simulink model "lab_cc_controlador"  (R2015a)
settings: Solver=ode45  StartTime=0.0  StopTime=40  RelTol=1e-6
values from neighbouring files (symbols this model uses):
  A = [2.8883370741 1 0 0 0 -2.75968400411 0 1 0 0 0.525095601237 0 ... (25 elements, 5x5)]    [model_matrix_data424.mat]
  B = [1 0 0 0 0]    [model_matrix_data424.mat]
  C = [-0.0748175001742 0.149096420272 0 0 0]    [model_matrix_data424.mat]
  D = 0    [model_matrix_data424.mat]
  N = Ny+K*Nx    [lab4script.m]    (also in test_different_R.m; teste_sistema_real.m)
  Ts = 0.02    [lab4script.m]    (also in test_different_R.m; teste_sistema_real.m)
undefined symbols (not defined in the file or in its folder): K, M
settings Model: Creator=Margarida  LastModifiedBy=Margarida

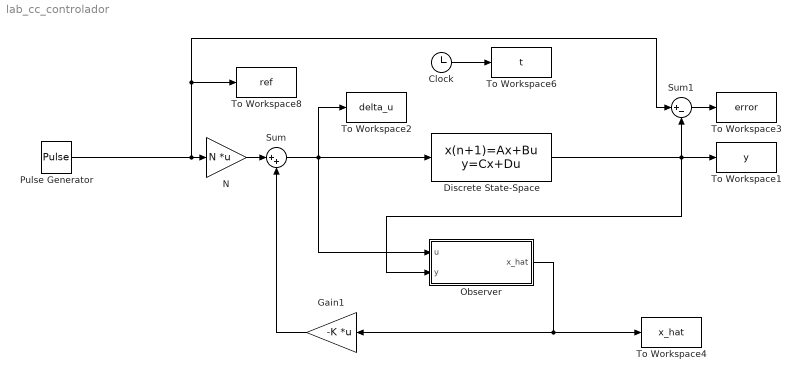
== system lab_cc_controlador ==
  Clock : Clock
  Discrete State-Space : DiscreteStateSpace  A=A  B=B  C=C  D=D  SampleTime=Ts
  Gain1 : Gain  Gain=-K  Multiplication=Matrix(K*u)
  N : Gain  Gain=N  Multiplication=Matrix(K*u)
  Observer : Subsystem
  Pulse Generator : DiscretePulseGenerator  Period=800  PulseWidth=400  SampleTime=Ts
  Sum : Sum  Inputs=|++
  Sum1 : Sum  Inputs=|+-
  To Workspace1 : ToWorkspace  VariableName=y  SampleTime=Ts
  To Workspace2 : ToWorkspace  VariableName=delta_u  SampleTime=Ts
  To Workspace3 : ToWorkspace  VariableName=error  SampleTime=Ts
  To Workspace4 : ToWorkspace  VariableName=x_hat  SampleTime=Ts
  To Workspace6 : ToWorkspace  VariableName=t  SampleTime=Ts
  To Workspace8 : ToWorkspace  VariableName=ref  SampleTime=Ts
  wires:
  Discrete State-Space/1 -> Observer/2(y), To Workspace1/1, Sum1/2
  Observer/1(x_hat) -> Gain1/1, To Workspace4/1
  Gain1/1 -> Sum/2
  Sum/1 -> To Workspace2/1, Observer/1(u), Discrete State-Space/1
  Clock/1 -> To Workspace6/1
  N/1 -> Sum/1
  Pulse Generator/1 -> To Workspace8/1, Sum1/1, N/1
  Sum1/1 -> To Workspace3/1

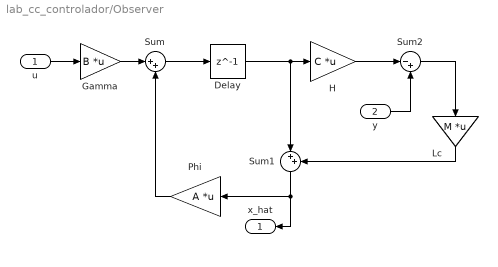
== system lab_cc_controlador/Observer ==
  u : Inport
  y : Inport  Port=2
  Delay : Delay  DelayLength=1  InitialCondition=0  SampleTime=Ts
  Gamma : Gain  Gain=B  Multiplication=Matrix(K*u)
  H : Gain  Gain=C  Multiplication=Matrix(K*u)
  Lc : Gain  Gain=M  Multiplication=Matrix(K*u)
  "Phi " : Gain  Gain=A  Multiplication=Matrix(K*u)
  Sum : Sum  Inputs=|++
  Sum1 : Sum  Inputs=|++
  Sum2 : Sum  Inputs=|-+
  x_hat : Outport
  wires:
  Gamma/1 -> Sum/1
  Sum/1 -> Delay/1
  Delay/1 -> Sum1/1, H/1
  "Phi "/1 -> Sum/2
  Sum1/1 -> x_hat/1, "Phi "/1
  H/1 -> Sum2/1
  Sum2/1 -> Lc/1
  Lc/1 -> Sum1/2
  u/1 -> Gamma/1
  y/1 -> Sum2/2
